simulink model "rtwdemo_atomic"  (Simulink 6.0)
settings: Solver=FixedStepDiscrete  StartTime=0.0  StopTime=10.0  RelTol=1e-3
undefined symbols (not defined in the file or in its folder): DiscIntNeverNeededParam
libraries: rtwdemowidgets x2
settings Model: Creator=The MathWorks Inc.  LastModifiedBy=batserve  ExtModeAutoUpdateStatusClock=off
settings DataIOCC: SaveOutput=off  SaveTime=off  SignalLoggingName=sigsOut
settings OptimizationCC: InlineParams=on  EnforceIntegerDowncast=off  StateBitsets=on  DataBitsets=on  UseTempVars=on
settings DebuggingCC: CheckExecutionContextPreStartOutputMsg=on  CheckExecutionContextRuntimeOutputMsg=on  SolverPrmCheckMsg=none
settings RTWCC: TLCOptions=-p0 -aWarnNonSaturatedBlocks=0  GenerateReport=on  RTWVerbose=off  ProcessScript=grt_make_rtw_hook  LaunchReport=on
settings CodeAppCC: ForceParamTrailComments=on  PrefixModelToSubsysFcnNames=off
settings GRTTargetCC: MatFileLogging=off

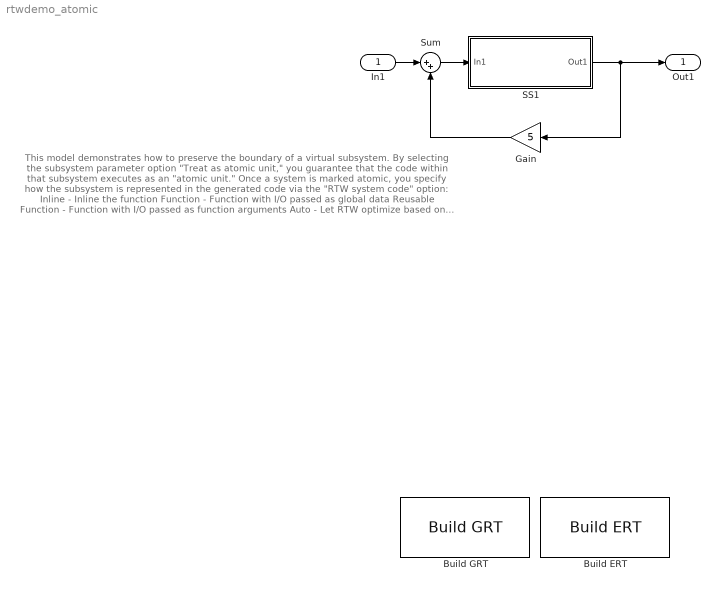
== system rtwdemo_atomic ==
  note: This model demonstrates how to preserve the boundary of a virtual subsystem.  By selecting the subsystem
      | parameter option "Treat as atomic unit," you guarantee that the code within that subsystem executes as
      | an "atomic unit."  Once a system is marked atomic, you specify how the subsystem is represented in the
      | generated code via the "RTW system code" option:
      |
      | Inline            - Inline the function
      | Function          - Function with I/O passed as global data
      | Reusable Function - Function with I/O passed as function arguments
      | Auto              - Let RTW optimize based on context
      |
      | The function name is controlled with the "RTW function name" option.  Here, SS1 is configured as
      | "Function" with function name "myfun."
      |
      | Note how Simulink and Real-Time Workshop avoid an "artificial" algebraic loop when the subsystem is made
      | atomic!  This is done by splitting up the output and update sections of the system into two functions
      | myfun (output) and myfun_update (update).  In the case that algebraic loop avoidance is not necessary,
      | there is a single step function.  For example, you will see a single step function "myfun" when the
      | feedback loop is removed in this example.
  In1 : Inport  Port=1  LatchInput=off
  Build ERT : rtwdemowidgets/Build ERT  attrib_overrides={}
  Build GRT : rtwdemowidgets/Build GRT  attrib_overrides={}
  Gain : Gain  Orientation=left  Gain=5  SaturateOnIntegerOverflow=on
  SS1 : Subsystem  TreatAsAtomicUnit=on  PropExecContextAcrossSSBoundary=on  RTWFcnName=myfun  RTWFileName=myfile
      settings: RTWFcnNameOpts=User specified
  Sum : Sum  Inputs=|++
  Out1 : Outport
  wires:
  Sum/1 -> SS1/1(In1)
  In1/1 -> Sum/1
  SS1/1(Out1) -> Out1/1, Gain/1
  Gain/1 -> Sum/2

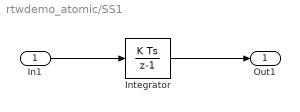
== system rtwdemo_atomic/SS1 ==
  In1 : Inport  Port=1  LatchInput=off
  Integrator : DiscreteIntegrator  ICPrevOutput=DiscIntNeverNeededParam  ICPrevScaledInput=DiscIntNeverNeededParam
  Out1 : Outport
  wires:
  In1/1 -> Integrator/1
  Integrator/1 -> Out1/1
